simulink model "TestforDzZOH"  (R2019b)
settings: Solver=FixedStepAuto  StartTime=0.0  StopTime=50  FixedStep=0.2  RelTol=1e-3
settings Model: Creator=Administrator  LastModifiedBy=Administrator

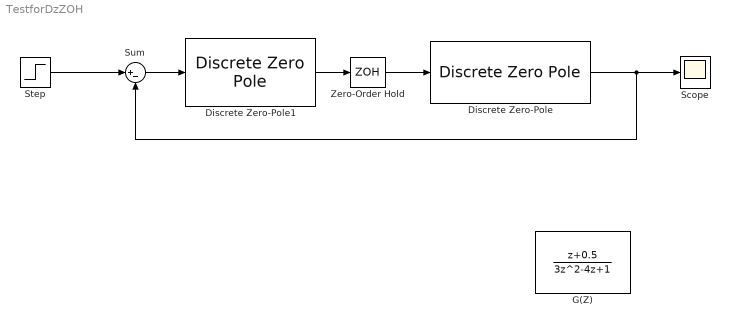
== system TestforDzZOH ==
  Discrete Zero-Pole : DiscreteZeroPole  Zeros=[]  Poles=[0 0.5]  Gain=1  SampleTime=-1
  Discrete Zero-Pole1 : DiscreteZeroPole  Zeros=[0]  Poles=[1]  Gain=0.25  SampleTime=-1
  G(Z) : DiscreteTransferFcn  Numerator=[1 0.5]  Denominator=[3 -4 1]
  Scope : Scope
  Step : Step  Time=0  SampleTime=0
  Sum : Sum  Inputs=|+-
  Zero-Order Hold : ZeroOrderHold  SampleTime=0.2
  wires:
  Step/1 -> Sum/1
  Discrete Zero-Pole/1 -> Sum/2, Scope/1
  Zero-Order Hold/1 -> Discrete Zero-Pole/1
  Sum/1 -> Discrete Zero-Pole1/1
  Discrete Zero-Pole1/1 -> Zero-Order Hold/1
